simulink model "A_2_10_FlightModel"  (R2024b)
settings: Solver=ode4  StartTime=0.0  StopTime=inf  FixedStep=(1/30)/10  RelTol=1e-3
values from neighbouring files (symbols this model uses):
  g = 9.81    [ParameterInSI.m]
  pitch = 0    [start.m]
  roll = 0    [start.m]
  throtle = 0    [start.m]
  yaw = 0    [start.m]
undefined symbols (not defined in the file or in its folder): ft, INI, m, s
libraries: aerolibconvert2 x5, aerolibasang x4, aerolibanimutils x2, aerolibfltsims x2, aerolibatmos2 x1, shared6dof x1
settings Model: Creator=the-main  LastModifiedBy=the_main

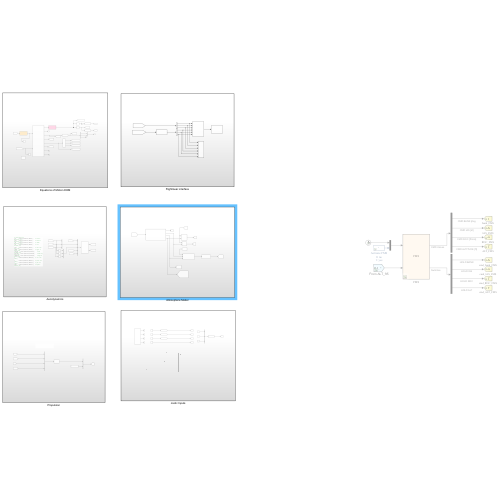
[thumbnail: Simulink's stored preview of the top-level diagram]
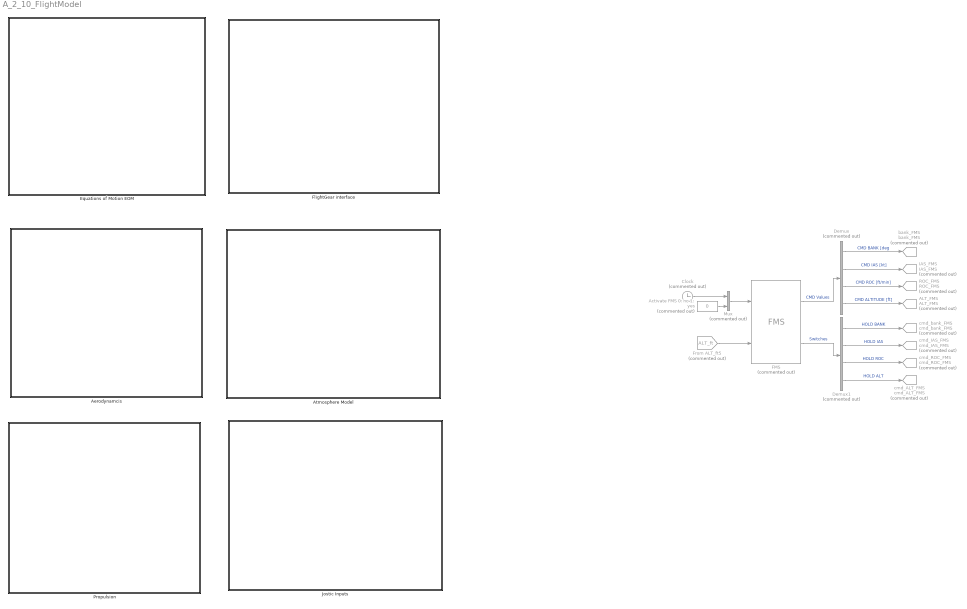
== system A_2_10_FlightModel ==
  ALT_FMS : Goto  Commented=on  GotoTag=ALT_FMS  TagVisibility=global
  Activate FMS 0: no 1: yes : Constant  Commented=on  Value=0
  Aerodynamcis : Subsystem
  Atmosphere Model : Subsystem
  Clock : Clock  Commented=on
  Demux : Demux  Commented=on
  Demux1 : Demux  Commented=on
  Equations of Motion EOM : Subsystem
  FMS : M-S-Function  Commented=on  FunctionName=FMS
  FlightGear interface : Subsystem
  From ALT_ft5 : From  Commented=on  GotoTag=ALT_ft  TagVisibility=global
  IAS_FMS : Goto  Commented=on  GotoTag=IAS_FMS  TagVisibility=global
  Jostic Inputs : Subsystem
  Mux : Mux  Commented=on  Inputs=2
  Propulsion : Subsystem
  ROC_FMS : Goto  Commented=on  GotoTag=ROC_FMS  TagVisibility=global
  bank_FMS : Goto  Commented=on  GotoTag=bank_FMS  TagVisibility=global
  cmd_ALT_FMS : Goto  Commented=on  GotoTag=cmd_ALT_FMS  TagVisibility=global
  cmd_IAS_FMS : Goto  Commented=on  GotoTag=cmd_IAS_FMS  TagVisibility=global
  cmd_ROC_FMS : Goto  Commented=on  GotoTag=cmd_ROC_FMS  TagVisibility=global
  cmd_bank_FMS : Goto  Commented=on  GotoTag=cmd_bank_FMS  TagVisibility=global
  wires:
  Demux/1 -> bank_FMS/1  "CMD BANK [deg"
  Demux1/4 -> cmd_ALT_FMS/1  "HOLD ALT"
  FMS/2 -> Demux1/1  "Switches"
  Mux/1 -> FMS/1
  From ALT_ft5/1 -> FMS/2
  Activate FMS 0: no 1: yes/1 -> Mux/2
  Demux1/3 -> cmd_ROC_FMS/1  "HOLD ROC"
  Demux1/1 -> cmd_bank_FMS/1  "HOLD BANK"
  Demux/4 -> ALT_FMS/1  "CMD ALTITUDE [ft]"
  Demux1/2 -> cmd_IAS_FMS/1  "HOLD IAS"
  Demux/3 -> ROC_FMS/1  "CMD ROC [ft/min]"
  Demux/2 -> IAS_FMS/1  "CMD IAS [kt]"
  FMS/1 -> Demux/1  "CMD Values"
  Clock/1 -> Mux/1

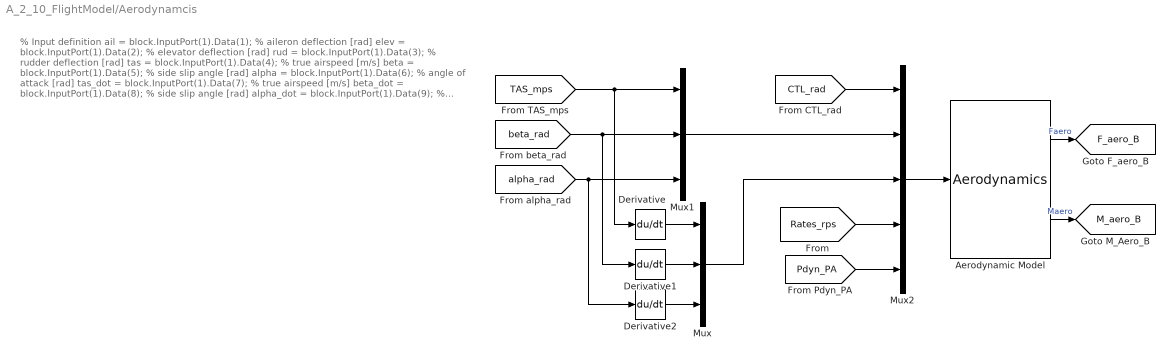
== system A_2_10_FlightModel/Aerodynamcis ==
  note: % Input definition
      | ail = block.InputPort(1).Data(1); % aileron deflection [rad]
      | elev = block.InputPort(1).Data(2); % elevator deflection [rad]
      | rud = block.InputPort(1).Data(3); % rudder deflection [rad]
      | tas = block.InputPort(1).Data(4); % true airspeed [m/s]
      | beta = block.InputPort(1).Data(5); % side slip angle [rad]
      | alpha = block.InputPort(1).Data(6); % angle of attack [rad]
      | tas_dot = block.InputPort(1).Data(7); % true airspeed [m/s]
      | beta_dot = block.InputPort(1).Data(8); % side slip angle [rad]
      | alpha_dot = block.InputPort(1).Data(9); % angle of attack [rad]
      | p = block.InputPort(1).Data(10); % roll rate [rad/s]
      | q = block.InputPort(1).Data(11); % pitch rate [rad/s]
      | r = block.InputPort(1).Data(12); % yaw rate [rad/s]
      | Pdyn = block.InputPort(1).Data(13); % dynamic pressure [Pa]
  Aerodynamic Model : M-S-Function  FunctionName=Aerodynamics
  Derivative : Derivative
  Derivative1 : Derivative
  Derivative2 : Derivative
  Mux : Mux  Inputs=3
  Mux1 : Mux  Inputs=3
  Mux2 : Mux  Inputs=5
  tag scope: F_aero_B=global, M_aero_B=global
  wires:
  [TAS_mps] -> Derivative/1, Mux1/1
  [Pdyn_PA] -> Mux2/5
  Mux1/1 -> Mux2/2
  Aerodynamic Model/1 -> [F_aero_B]  "Faero"
  Mux2/1 -> Aerodynamic Model/1
  [beta_rad] -> Mux1/2, Derivative1/1
  [CTL_rad] -> Mux2/1
  [alpha_rad] -> Mux1/3, Derivative2/1
  Aerodynamic Model/2 -> [M_aero_B]  "Maero"
  [Rates_rps] -> Mux2/4
  Derivative2/1 -> Mux/3
  Derivative1/1 -> Mux/2
  Derivative/1 -> Mux/1
  Mux/1 -> Mux2/3

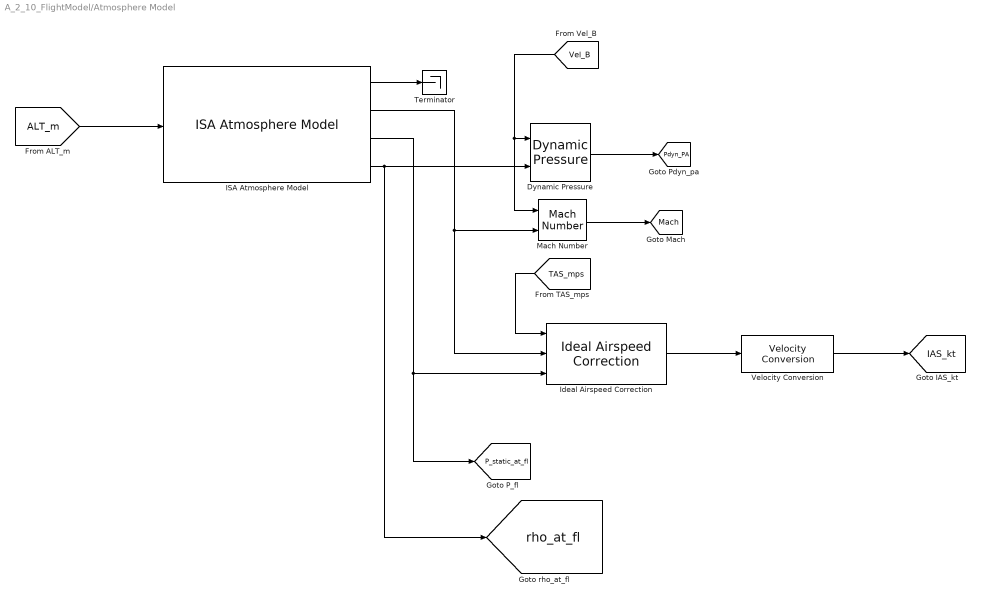
== system A_2_10_FlightModel/Atmosphere Model ==
  Dynamic Pressure : aerolibasang/Dynamic Pressure
  ISA Atmosphere Model : aerolibatmos2/ISA Atmosphere Model  useExtended=off  action=Warning  custom=off  viscosityOut=off  g=9.80665  gamma=1.4  R=287.0531  L=0.0065  h_trop=11000  h_strat=20000  rho0=1.225  P0=101325  T0=288.15  h0=0  S=110.4  Tref=273.15  muref=1.716e-5
  Ideal Airspeed Correction : aerolibasang/Ideal Airspeed Correction  units=Metric (MKS)  vel_in=TAS  vel_out_tas=EAS  vel_out_eas=TAS  vel_out_cas=TAS  method=Table Lookup  SubOnly=off  action=None
  Mach Number : aerolibasang/Mach Number
  Terminator : Terminator
  Velocity Conversion : aerolibconvert2/Velocity Conversion  IU=m/s  OU=kts
  tag scope: IAS_kt=global, Mach=global, P_static_at_fl=global, Pdyn_PA=global, rho_at_fl=global
  wires:
  Velocity Conversion/1 -> [IAS_kt]
  ISA Atmosphere Model/1 -> Terminator/1
  ISA Atmosphere Model/4 -> [rho_at_fl], Dynamic Pressure/2
  [Vel_B] -> Mach Number/1, Dynamic Pressure/1
  [ALT_m] -> ISA Atmosphere Model/1
  Mach Number/1 -> [Mach]
  Dynamic Pressure/1 -> [Pdyn_PA]
  ISA Atmosphere Model/3 -> [P_static_at_fl], Ideal Airspeed Correction/3
  [TAS_mps] -> Ideal Airspeed Correction/1
  ISA Atmosphere Model/2 -> Mach Number/2, Ideal Airspeed Correction/2
  Ideal Airspeed Correction/1 -> Velocity Conversion/1

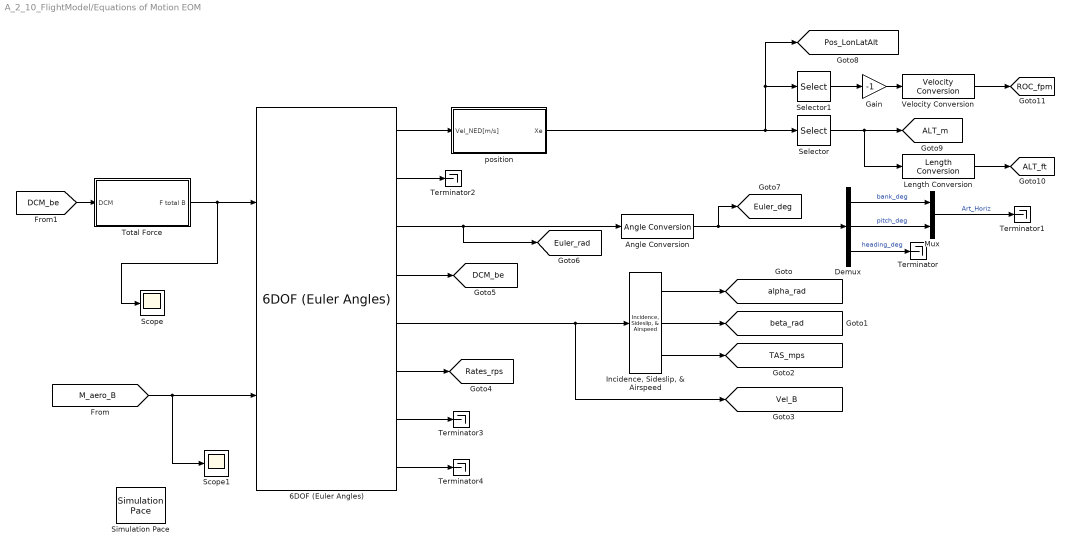
== system A_2_10_FlightModel/Equations of Motion EOM ==
  6DOF (Euler Angles) : shared6dof/6DOF (Euler Angles)  units=Metric (MKS)  mtype=Fixed  rep=Euler Angles  xme_0=[0 0 0]  Vm_0=INI.VELbod  eul_0=[0 0 0]  pm_0=[0 0 0]  mass_0=INI.mass  mass_e=0.5  mass_f=2.0  inertia=INI.Inertia  inertia_e=eye(3)  inertia_f=2*eye(3)  k_quat=1.0  vre_flag=on  abi_flag=off  aMode=0  xme_statename=''  Vm_statename=''  eul_statename=''  quat_statename=''  pm_statename=''  mass_statename=''
  Angle Conversion : aerolibconvert2/Angle Conversion  IU=rad  OU=deg
  Demux : Demux  Outputs=3
  Gain : Gain  Gain=-1
  "Incidence, Sideslip, & Airspeed" : aerolibasang/Incidence, Sideslip, & Airspeed
  Length Conversion : aerolibconvert2/Length Conversion  IU=m  OU=ft
  Mux : Mux  Inputs=2
  Scope : Scope
  Scope1 : Scope
  Selector : Selector  InputPortWidth=3  IndexOptions=Starting index (dialog)  Indices=3  OutputSizes=1
  Selector1 : Selector  InputPortWidth=3  IndexOptions=Starting index (dialog)  Indices=3  OutputSizes=1
  Simulation Pace : aerolibanimutils/Simulation Pace  SimulationPace=1  SleepMode=Auto  OutputPaceError=off  SampleTime=1/30
  Terminator{,1..4} (5 alike) : Terminator
  Total Force : Subsystem
  Velocity Conversion : aerolibconvert2/Velocity Conversion  IU=m/s  OU=ft/min
  position : Subsystem
  tag scope: ALT_ft=global, ALT_m=global, DCM_be=global, Euler_deg=global, Euler_rad=global, Pos_LonLatAlt=global, ROC_fpm=global, Rates_rps=global, TAS_mps=global, Vel_B=global, alpha_rad=global, beta_rad=global
  wires:
  6DOF (Euler Angles)/5 -> [Vel_B], "Incidence, Sideslip, & Airspeed"/1
  "Incidence, Sideslip, & Airspeed"/1 -> [alpha_rad]
  "Incidence, Sideslip, & Airspeed"/2 -> [beta_rad]
  "Incidence, Sideslip, & Airspeed"/3 -> [TAS_mps]
  6DOF (Euler Angles)/6 -> [Rates_rps]
  [M_aero_B] -> Scope1/1, 6DOF (Euler Angles)/2
  Total Force/1(F total B) -> 6DOF (Euler Angles)/1, Scope/1
  [DCM_be] -> Total Force/1(DCM)
  6DOF (Euler Angles)/4 -> [DCM_be]
  6DOF (Euler Angles)/3 -> Angle Conversion/1, [Euler_rad]
  Angle Conversion/1 -> Demux/1, [Euler_deg]
  Demux/1 -> Mux/1  "bank_deg"
  Demux/2 -> Mux/2  "pitch_deg"
  Mux/1 -> Terminator1/1  "Art_Horiz"
  6DOF (Euler Angles)/1 -> position/1(Vel_NED[m/s])
  Demux/3 -> Terminator/1  "heading_deg"
  6DOF (Euler Angles)/2 -> Terminator2/1
  position/1(Xe) -> Selector1/1, [Pos_LonLatAlt], Selector/1
  Selector/1 -> Length Conversion/1, [ALT_m]
  Length Conversion/1 -> [ALT_ft]
  Selector1/1 -> Gain/1
  Gain/1 -> Velocity Conversion/1
  Velocity Conversion/1 -> [ROC_fpm]
  6DOF (Euler Angles)/7 -> Terminator3/1
  6DOF (Euler Angles)/8 -> Terminator4/1

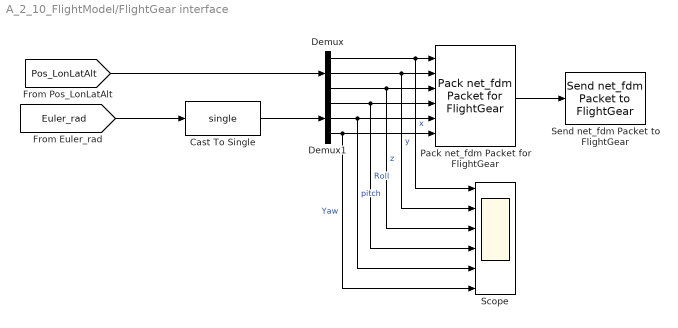
== system A_2_10_FlightModel/FlightGear interface ==
  Cast To Single : DataTypeConversion  OutDataTypeStr=single  SaturateOnIntegerOverflow=off  RndMeth=Floor
  Demux : Demux  Outputs=3
  Demux1 : Demux  Outputs=3
  Pack net_fdm Packet for FlightGear : aerolibfltsims/Pack net_fdm Packet for FlightGear  FlightGearVersion=v2019.1  ShowPositionAttitudeInputs=on  ShowVelocityAccelerationInputs=off  ShowControlSurfacePositionInputs=off  ShowEngineFuelInputs=off  ShowLandingGearInputs=off  ShowEnvironmentInputs=off  SampleTime=1/30  packetVersion=24
  Scope : Scope  NumInputPorts=6
  Send net_fdm Packet to FlightGear : aerolibfltsims/Send net_fdm Packet to FlightGear  DestinationIpAddress=127.0.0.1  DestinationPort=5502  LocalIpPort=-1  varLen=off  SampleTime=1/30
  wires:
  Pack net_fdm Packet for FlightGear/1 -> Send net_fdm Packet to FlightGear/1
  [Pos_LonLatAlt] -> Demux/1
  Demux/1 -> Scope/1, Pack net_fdm Packet for FlightGear/1  "x"
  Demux/2 -> Scope/2, Pack net_fdm Packet for FlightGear/2  "y"
  Demux/3 -> Scope/3, Pack net_fdm Packet for FlightGear/3  "z"
  [Euler_rad] -> Cast To Single/1
  Cast To Single/1 -> Demux1/1
  Demux1/1 -> Scope/4, Pack net_fdm Packet for FlightGear/4  "Roll"
  Demux1/2 -> Scope/5, Pack net_fdm Packet for FlightGear/5  "pitch"
  Demux1/3 -> Scope/6, Pack net_fdm Packet for FlightGear/6  "Yaw"

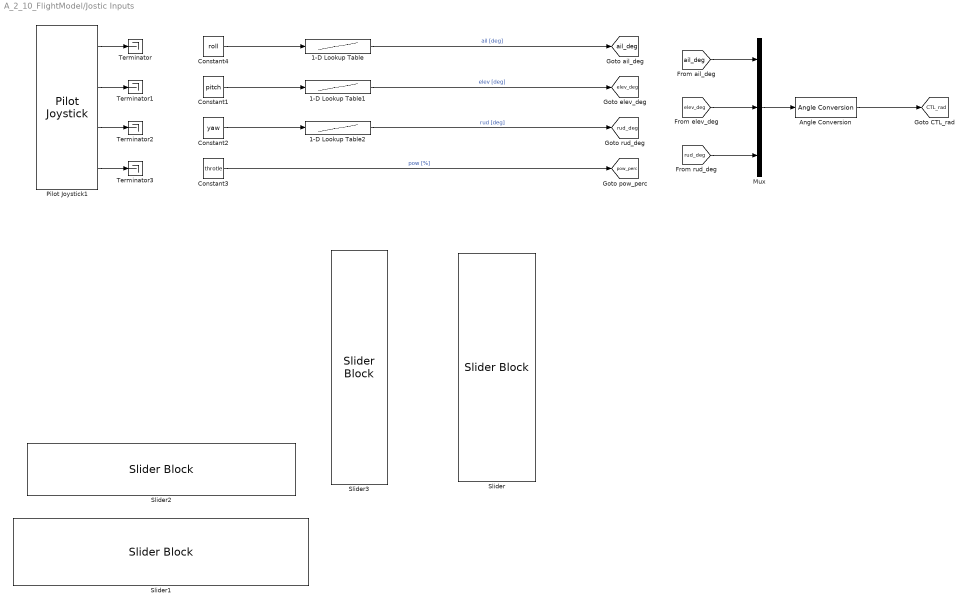
== system A_2_10_FlightModel/Jostic Inputs ==
  1-D Lookup Table : Lookup_n-D  NumberOfTableDimensions=1  BreakpointsForDimension1=[-5:5]  Table=tanh([-5:5])  InternalRulePriority=Speed  RndMeth=Simplest
  1-D Lookup Table1 : Lookup_n-D  NumberOfTableDimensions=1  BreakpointsForDimension1=[-5:5]  Table=tanh([-5:5])  InternalRulePriority=Speed  RndMeth=Simplest
  1-D Lookup Table2 : Lookup_n-D  NumberOfTableDimensions=1  BreakpointsForDimension1=[-5:5]  Table=tanh([-5:5])  InternalRulePriority=Speed  RndMeth=Simplest
  Angle Conversion : aerolibconvert2/Angle Conversion  IU=deg  OU=rad
  Constant1 : Constant  Value=pitch
  Constant2 : Constant  Value=yaw
  Constant3 : Constant  Value=throtle
  Constant4 : Constant  Value=roll
  Mux : Mux  Inputs=3
  Pilot Joystick1 : aerolibanimutils/Pilot Joystick  JoystickID=Joystick1  OutputConfiguration=FourAxis  SampleTime=1/30
  Slider : SliderBlock  ScaleMax=1
  Slider1 : SliderBlock  ScaleMin=-30  ScaleMax=30
  Slider2 : SliderBlock  ScaleMin=-30  ScaleMax=30
  Slider3 : SliderBlock  ScaleMin=-50  ScaleMax=50
  Terminator{,1..3} (4 alike) : Terminator
  tag scope: CTL_rad=global, ail_deg=global, elev_deg=global, pow_perc=global, rud_deg=global
  wires:
  Constant4/1 -> 1-D Lookup Table/1
  1-D Lookup Table1/1 -> [elev_deg]  "elev [deg]"
  [elev_deg] -> Mux/2
  [ail_deg] -> Mux/1
  1-D Lookup Table/1 -> [ail_deg]  "ail [deg]"
  Constant3/1 -> [pow_perc]  "pow [%]"
  Angle Conversion/1 -> [CTL_rad]
  Constant2/1 -> 1-D Lookup Table2/1
  Constant1/1 -> 1-D Lookup Table1/1
  [rud_deg] -> Mux/3
  1-D Lookup Table2/1 -> [rud_deg]  "rud [deg]"
  Mux/1 -> Angle Conversion/1
  Pilot Joystick1/1 -> Terminator/1
  Pilot Joystick1/2 -> Terminator1/1
  Pilot Joystick1/3 -> Terminator2/1
  Pilot Joystick1/4 -> Terminator3/1

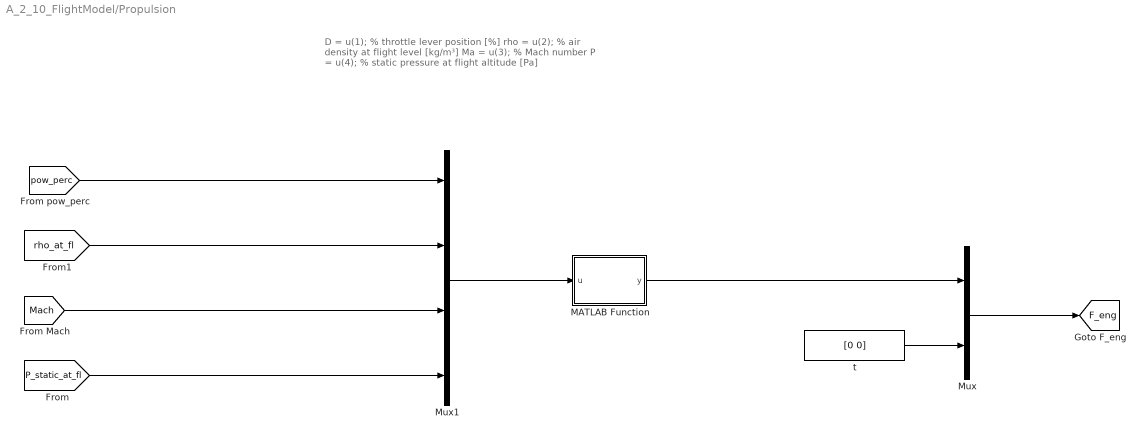
== system A_2_10_FlightModel/Propulsion ==
  note: D       = u(1);         % throttle lever position [%]
      | rho     = u(2);         % air density at flight level [kg/m³]
      | Ma      = u(3);         % Mach number
      | P       = u(4);         % static pressure at flight altitude [Pa]
  MATLAB Function : MATLAB Function  TreatAsAtomicUnit=on
  Mux : Mux  Inputs=2
  Mux1 : Mux
  t : Constant  Value=[0 0]
  tag scope: F_eng=global
  wires:
  Mux/1 -> [F_eng]
  t/1 -> Mux/2
  MATLAB Function/1(y) -> Mux/1
  [pow_perc] -> Mux1/1
  [rho_at_fl] -> Mux1/2
  Mux1/1 -> MATLAB Function/1(u)
  [Mach] -> Mux1/3
  [P_static_at_fl] -> Mux1/4

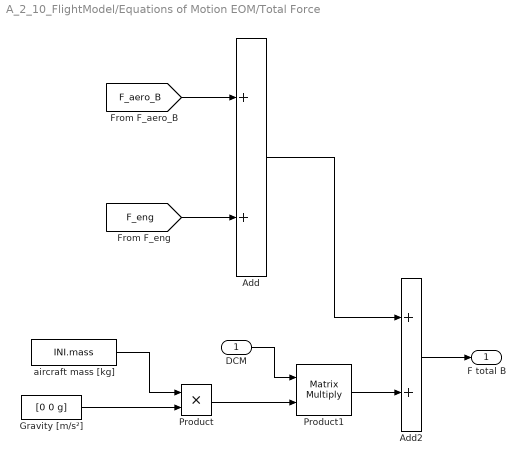
== system A_2_10_FlightModel/Equations of Motion EOM/Total Force ==
  DCM : Inport
  Add : Sum
  Add2 : Sum
  Gravity [m/s²] : Constant  Value=[0 0 g]
  Product : Product
  Product1 : Product  Multiplication=Matrix(*)
  aircraft mass [kg] : Constant  Value=INI.mass
  F total B : Outport  VectorParamsAs1DForOutWhenUnconnected=off
  wires:
  Add/1 -> Add2/1
  Gravity [m/s²]/1 -> Product/2
  Product1/1 -> Add2/2
  Add2/1 -> F total B/1
  Product/1 -> Product1/2
  aircraft mass [kg]/1 -> Product/1
  DCM/1 -> Product1/1
  [F_eng] -> Add/2
  [F_aero_B] -> Add/1

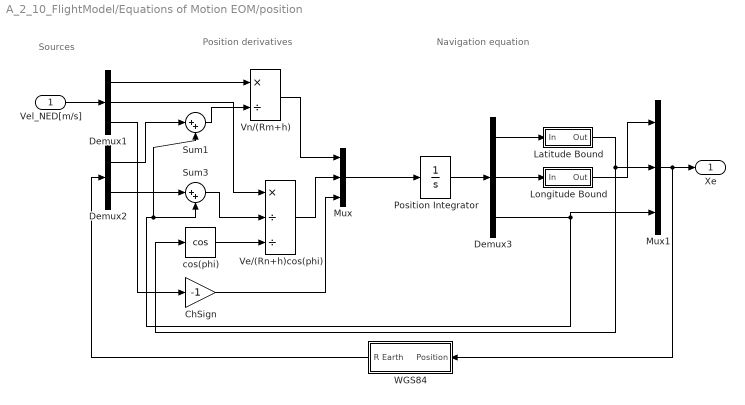
== system A_2_10_FlightModel/Equations of Motion EOM/position ==
  note: Navigation equation
  note: Position derivatives
  note: Sources
  Vel_NED[m/s] : Inport
  ChSign : Gain  Gain=-1  SaturateOnIntegerOverflow=on  OutDataTypeStr=Inherit: Same as input  ParamDataTypeStr=Inherit: Same as input
  Demux1 : Demux  Outputs=3
      settings: DisplayOption=none
  Demux2 : Demux  Outputs=2
      settings: DisplayOption=none
  Demux3 : Demux  Outputs=3
      settings: DisplayOption=none
  Latitude Bound : Subsystem
  Longitude Bound : Subsystem
  Mux : Mux  Inputs=3
  Mux1 : Mux  Inputs=3
  Position Integrator : Integrator  InitialCondition=INI.POS
  Sum1 : Sum  Inputs=|++
  Sum3 : Sum  Inputs=|++
  Ve/(Rn+h)cos(phi) : Product  Inputs=*//  InputSameDT=on  SaturateOnIntegerOverflow=on  OutDataTypeStr=Inherit: Same as first input
  Vn/(Rm+h) : Product  Inputs=*/  InputSameDT=on  SaturateOnIntegerOverflow=on  OutDataTypeStr=Inherit: Same as first input
  WGS84 : Subsystem
  cos(phi) : Trigonometry  Operator=cos
  Xe : Outport  VectorParamsAs1DForOutWhenUnconnected=off
  wires:
  Longitude Bound/1(Out) -> Mux1/1
  Mux1/1 -> Xe/1, WGS84/1(Position)
  cos(phi)/1 -> Ve/(Rn+h)cos(phi)/3
  Demux3/1 -> Latitude Bound/1(In)
  ChSign/1 -> Mux/3
  Latitude Bound/1(Out) -> cos(phi)/1, Mux1/2
  Vn/(Rm+h)/1 -> Mux/1
  Demux1/2 -> Ve/(Rn+h)cos(phi)/1
  Demux1/1 -> Vn/(Rm+h)/1
  Vel_NED[m/s]/1 -> Demux1/1
  Demux1/3 -> ChSign/1
  Demux3/2 -> Longitude Bound/1(In)
  Demux3/3 -> Mux1/3, Sum3/2, Sum1/2
  Ve/(Rn+h)cos(phi)/1 -> Mux/2
  WGS84/1(R Earth) -> Demux2/1
  Sum1/1 -> Vn/(Rm+h)/2
  Demux2/1 -> Sum1/1
  Demux2/2 -> Sum3/1
  Sum3/1 -> Ve/(Rn+h)cos(phi)/2
  Position Integrator/1 -> Demux3/1
  Mux/1 -> Position Integrator/1

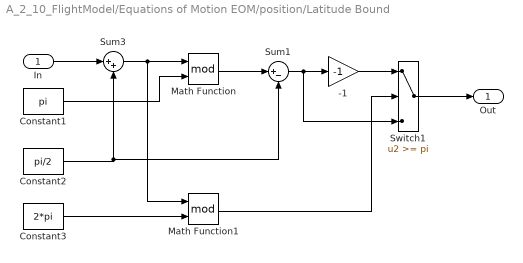
== system A_2_10_FlightModel/Equations of Motion EOM/position/Latitude Bound ==
  In : Inport
  -1 : Gain  Gain=-1  SaturateOnIntegerOverflow=on  OutDataTypeStr=Inherit: Same as input  ParamDataTypeStr=Inherit: Same as input
  Constant1 : Constant  Value=pi
  Constant2 : Constant  Value=pi/2
  Constant3 : Constant  Value=2*pi
  Math Function : Math  Operator=mod  SignedPower=on
  Math Function1 : Math  Operator=mod  SignedPower=on
  Sum1 : Sum  Inputs=|+-
  Sum3 : Sum  Inputs=|++
  Switch1 : Switch  Threshold=pi  SaturateOnIntegerOverflow=off  InputSameDT=off
  Out : Outport  VectorParamsAs1DForOutWhenUnconnected=off
  wires:
  -1/1 -> Switch1/1
  Switch1/1 -> Out/1
  Math Function/1 -> Sum1/1
  Sum1/1 -> Switch1/3, -1/1
  Constant3/1 -> Math Function1/2
  Constant2/1 -> Sum1/2, Sum3/2
  Constant1/1 -> Math Function/2
  In/1 -> Sum3/1
  Math Function1/1 -> Switch1/2
  Sum3/1 -> Math Function1/1, Math Function/1

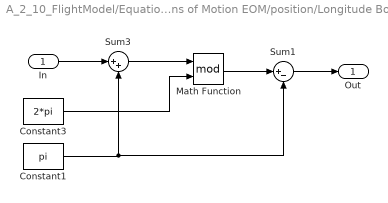
== system A_2_10_FlightModel/Equations of Motion EOM/position/Longitude Bound ==
  In : Inport
  Constant1 : Constant  Value=pi
  Constant3 : Constant  Value=2*pi
  Math Function : Math  Operator=mod  SignedPower=on
  Sum1 : Sum  Inputs=|+-
  Sum3 : Sum  Inputs=|++
  Out : Outport  VectorParamsAs1DForOutWhenUnconnected=off
  wires:
  Sum3/1 -> Math Function/1
  In/1 -> Sum3/1
  Constant1/1 -> Sum1/2, Sum3/2
  Constant3/1 -> Math Function/2
  Math Function/1 -> Sum1/1
  Sum1/1 -> Out/1

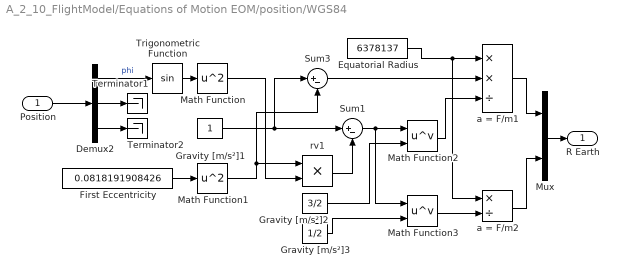
== system A_2_10_FlightModel/Equations of Motion EOM/position/WGS84 ==
  Position : Inport
  Demux2 : Demux  Outputs=3
  Equatorial Radius : Constant  Value=6378137
  First Eccentricity : Constant  Value=0.0818191908426
  Gravity [m/s²]1 : Constant
  Gravity [m/s²]2 : Constant  Value=3/2
  Gravity [m/s²]3 : Constant  Value=1/2
  Math Function : Math  Operator=square  SignedPower=on
  Math Function1 : Math  Operator=square  SignedPower=on
  Math Function2 : Math  Operator=pow  SignedPower=on
  Math Function3 : Math  Operator=pow  SignedPower=on
  Mux : Mux  Inputs=2
  Sum1 : Sum  Inputs=|+-
  Sum3 : Sum  Inputs=|+-
  Terminator1 : Terminator
  Terminator2 : Terminator
  Trigonometric Function : Trigonometry
  a = F/m1 : Product  Inputs=**/
  a = F/m2 : Product  Inputs=*/
  rv1 : Product
  R Earth : Outport  VectorParamsAs1DForOutWhenUnconnected=off
  wires:
  Gravity [m/s²]2/1 -> Math Function2/2
  a = F/m2/1 -> Mux/2
  Gravity [m/s²]3/1 -> Math Function3/2
  Math Function3/1 -> a = F/m2/2
  First Eccentricity/1 -> Math Function1/1
  Math Function1/1 -> Sum3/2, rv1/1
  Trigonometric Function/1 -> Math Function/1
  rv1/1 -> Sum1/2
  Sum1/1 -> Math Function3/1, Math Function2/1
  Position/1 -> Demux2/1
  Demux2/1 -> Trigonometric Function/1  "phi"
  Demux2/3 -> Terminator2/1
  Demux2/2 -> Terminator1/1
  a = F/m1/1 -> Mux/1
  Math Function/1 -> rv1/2
  Math Function2/1 -> a = F/m1/3
  Equatorial Radius/1 -> a = F/m2/1, a = F/m1/1
  Sum3/1 -> a = F/m1/2
  Gravity [m/s²]1/1 -> Sum1/1, Sum3/1
  Mux/1 -> R Earth/1

== matlab function A_2_10_FlightModel/Propulsion/MATLAB Function ==
  data: u input; y output
function y = fcn(u)

%  Parameters
Fmax    = 2500;         % maximum engine thrust [N]
mu      = 3.2;       	% engine bypass ratio
rho_0   = 1.225;     	% air density at sea level [kg/m³]
P_0     = 101325;     	% static air pressure at sea level [Pa]

% Variables 
D       = u(1);         % throttle lever position [%]  
rho     = u(2);         % air density at flight level [kg/m³]
Ma      = u(3);         % Mach number
P       = u(4);         % static pressure at flight altitude [Pa]

% Code
% engine thrust [N]
F = Fmax * (D / 100) * (rho / rho_0) * exp(-0.35 * Ma * (P / P_0) * sqrt(mu));

y = F;
